simulink model "speed_ctl_tf_sim"  (R2023a)
settings: configuration reference "config" (kept outside this file)
model workspace (MATLAB code in the model file + MAT data in the model file):
  cmdLim = Simulink.Parameter
  cmdLim.Value = 15
  cmdLim.Description = 'Limit for controlling the maximum surface command angle.'
  cmdLim.Min = 0
  cmdLim.Max = 90
  cmdLim.DocUnits = 'deg'
  dispGain = Simulink.Parameter
  dispGain.Value = 0.75
  dispGain.Description = 'Gain applied to the displacement error.'
  dispGain.Min = 0
  dispGain.Max = []
  dispGain.DocUnits = 'deg/sec/deg'
  dispLim = Simulink.Parameter
  dispLim.Value = 30
  dispLim.Description = 'Limit for controlling the maximum commanded angle.'
  dispLim.Min = 0
  dispLim.Max = 180
  dispLim.DocUnits = 'deg'
  intGain = Simulink.Parameter
  intGain.Value = 0.5
  intGain.Description = 'Gain applied to the integral error.'
  intGain.Min = 0
  intGain.Max = []
  intGain.DocUnits = 'deg/sec/deg/sec'
  intLim = Simulink.Parameter
  intLim.Value = 5
  intLim.Description = 'Limit for controlling the maximum commanded angle.'
  intLim.Min = 0
  intLim.Max = 90
  intLim.DocUnits = 'deg'
  rateGain = Simulink.Parameter
  rateGain.Value = 2
  rateGain.Description = 'Gain applied to the rate error.'
  rateGain.Min = 0
  rateGain.Max = []
  rateGain.DocUnits = 'deg/deg/sec'
  rateLim = Simulink.Parameter
  rateLim.Value = 6
  rateLim.Description = 'Limit for controlling the maximum commanded angle.'
  rateLim.Min = 0
  rateLim.Max = 180
  rateLim.DocUnits = 'deg/sec'
  hdgGain = Simulink.Parameter
  hdgGain.Value = 0.015
  b = Simulink.Parameter
  b.Value = 0.001
  b.DataType = 'single'
  b.Complexity = 'real'
  b.Dimensions = [1 1]
  current_ctl_bw_rad_s = Simulink.Parameter
  current_ctl_bw_rad_s.Value = 6666.7
  current_ctl_bw_rad_s.Description = '电流环设计带宽'
  current_ctl_bw_rad_s.DataType = 'single'
  current_ctl_bw_rad_s.Complexity = 'real'
  current_ctl_bw_rad_s.Dimensions = [1 1]
  delta = Simulink.Parameter
  delta.Value = 6
  delta.Description = '速度环阻尼因子'
  delta.DataType = 'double'
  delta.Complexity = 'real'
  delta.Dimensions = [1 1]
  dt = Simulink.Parameter
  dt.Value = 1e-05
  dt.DataType = 'single'
  dt.Complexity = 'real'
  dt.Dimensions = [1 1]
  fc = Simulink.Parameter
  fc.Value = 0.001
  fc.DataType = 'single'
  fc.Complexity = 'real'
  fc.Dimensions = [1 1]
  flux = Simulink.Parameter
  flux.Value = 0.0083
  flux.DataType = 'single'
  flux.Complexity = 'real'
  flux.Dimensions = [1 1]
  fs = Simulink.Parameter
  fs.Value = 10000
  fs.Description = '位置环 速度环执行频率'
  fs.DataType = 'single'
  fs.Complexity = 'real'
  fs.Dimensions = [1 1]
  iq_max = Simulink.Parameter
  iq_max.Value = 30
  iq_max.DataType = 'double'
  iq_max.Complexity = 'real'
  iq_max.Dimensions = [1 1]
  j = Simulink.Parameter
  j.Value = 0.0115
  j.DataType = 'single'
  j.Complexity = 'real'
  j.Dimensions = [1 1]
  j_inv = Simulink.Parameter
  j_inv.Value = 86.9565217391
  j_inv.DataType = 'single'
  j_inv.Complexity = 'real'
  j_inv.Dimensions = [1 1]
  kt = Simulink.Parameter
  kt.Value = 0.05
  kt.Description = '转矩常数 N*M/A'
  kt.DataType = 'single'
  kt.Complexity = 'real'
  kt.Dimensions = [1 1]
  ld = Simulink.Parameter
  ld.Value = 0.00059
  ld.DataType = 'single'
  ld.Complexity = 'real'
  ld.Dimensions = [1 1]
  ld_inv = Simulink.Parameter
  ld_inv.Value = 1694.91525424
  ld_inv.DataType = 'single'
  ld_inv.Complexity = 'real'
  ld_inv.Dimensions = [1 1]
  lq = Simulink.Parameter
  lq.Value = 0.00059
  lq.DataType = 'single'
  lq.Complexity = 'real'
  lq.Dimensions = [1 1]
  lq_inv = Simulink.Parameter
  lq_inv.Value = 1694.91525424
  lq_inv.DataType = 'single'
  lq_inv.Complexity = 'real'
  lq_inv.Dimensions = [1 1]
  pn = Simulink.Parameter
  pn.Value = 4
  pn.DataType = 'single'
  pn.Complexity = 'real'
  pn.Dimensions = [1 1]
  r = Simulink.Parameter
  r.Value = 1.02
  r.DataType = 'single'
  r.Complexity = 'real'
  r.Dimensions = [1 1]
  tc = Simulink.Parameter
  tc.Value = 5e-05
  tc.Description = '电流环运行频率用来设定综合仿真的参数'
  tc.DataType = 'double'
  tc.Complexity = 'real'
  tc.Dimensions = [1 1]
  tp = Simulink.Parameter
  tp.Value = 0.0001
  tp.Description = '位置环速度环执行周期'
  tp.DataType = 'double'
  tp.Complexity = 'real'
  tp.Dimensions = [1 1]
  ts = Simulink.Parameter
  ts.Value = 1e-05
  ts.Description = '模型仿真的周期 s'
  ts.DataType = 'double'
  ts.Complexity = 'real'
  ts.Dimensions = [1 1]
  wn = Simulink.Parameter
  wn.Value = 9434
  wn.DataType = 'double'
  wn.Complexity = 'real'
  wn.Dimensions = [1 1]
undefined symbols (not defined in the file): DiscIntNeverNeededParam
settings Model: RequirementInfo={} %GIDa_fe9045fd_0412_4b6e_8206_617cc20e6fde  DataDictionary=model_config.sldd  ParameterArgumentNames=b,current_ctl_bw_rad_s,dt,fc,flux,fs,j,j_inv,kt,ld,ld_inv,lq,lq_inv,pn,r  Creator=Administrator  LastModifiedBy=Administrator
settings ConfigSetRef: SourceName=config

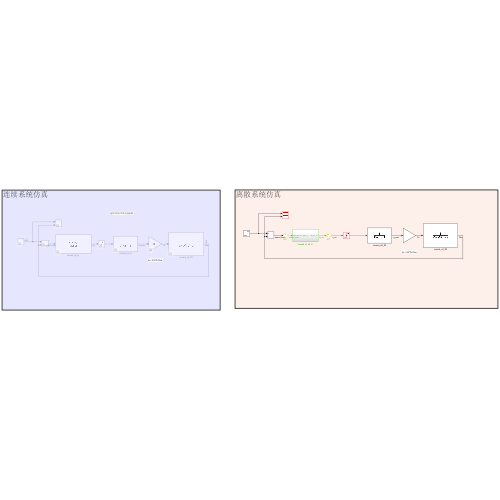
[thumbnail: Simulink's stored preview of the top-level diagram]
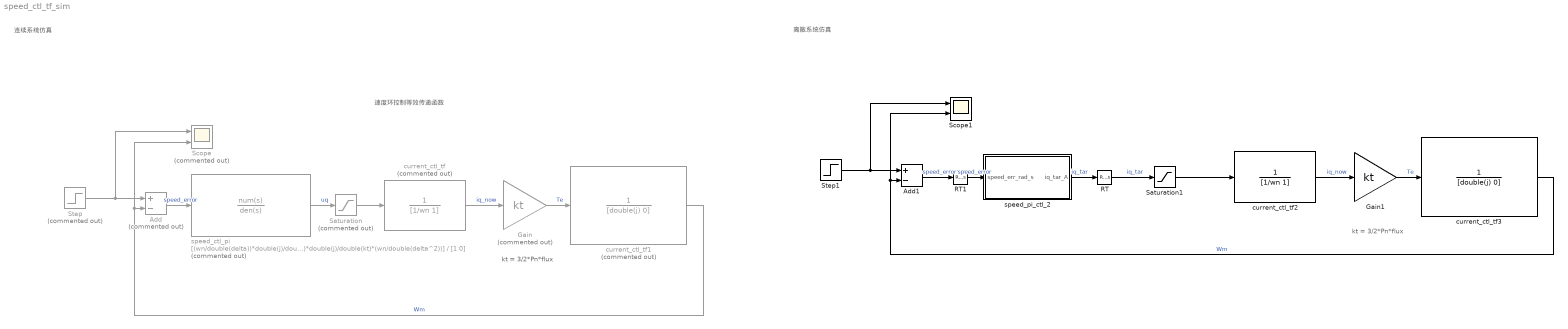
== system speed_ctl_tf_sim ==
  note: 速度环控制等效传递函数
  note: kt = 3/2*Pn*flux
  note: 离散系统仿真
  note: 连续系统仿真
  note: kt = 3/2*Pn*flux
  Add : Sum  Commented=on  Inputs=+-
  Add1 : Sum  Inputs=+-
  Gain : Gain  Commented=on  Gain=kt
  Gain1 : Gain  Gain=kt
  RT : RateTransition  OutPortSampleTime=1e-05
  RT1 : RateTransition  OutPortSampleTime=0.0001
  Saturation : Saturate  Commented=on  UpperLimit=iq_max  LowerLimit=-iq_max
  Saturation1 : Saturate  UpperLimit=iq_max  LowerLimit=-iq_max
  Scope : Scope  Commented=on  NumInputPorts=2
  Scope1 : Scope  NumInputPorts=2
  Step : Step  Commented=on  SampleTime=0
  Step1 : Step  SampleTime=0
  current_ctl_tf : TransferFcn  Commented=on  Denominator=[1/wn 1]
  current_ctl_tf1 : TransferFcn  Commented=on  Denominator=[double(j) 0]
  current_ctl_tf2 : TransferFcn  Denominator=[1/wn 1]
  current_ctl_tf3 : TransferFcn  Denominator=[double(j) 0]
  speed_ctl_pi : TransferFcn  Commented=on  Numerator="[(wn/double(delta))*double(j)/double(kt)    (wn/double(delta))*double(j)/double(kt)*(wn/double(delta^2))]"  Denominator=[1 0]
  speed_pi_ctl_2 : Subsystem  SystemSampleTime=10e-5
  wires:
  current_ctl_tf/1 -> Gain/1  "iq_now"
  Gain/1 -> current_ctl_tf1/1  "Te"
  speed_ctl_pi/1 -> Saturation/1  "uq"
  Add/1 -> speed_ctl_pi/1  "speed_error"
  Step/1 -> Scope/1, Add/1
  current_ctl_tf1/1 -> Scope/2, Add/2  "Wm"
  Step1/1 -> Scope1/1, Add1/1
  current_ctl_tf3/1 -> Scope1/2, Add1/2  "Wm"
  Add1/1 -> RT1/1  "speed_error"
  speed_pi_ctl_2/1(iq_tar_A) -> RT/1  "iq_tar"
  Gain1/1 -> current_ctl_tf3/1  "Te"
  current_ctl_tf2/1 -> Gain1/1  "iq_now"
  RT/1 -> Saturation1/1  "iq_tar"
  RT1/1 -> speed_pi_ctl_2/1(speed_err_rad_s)  "speed_error"
  Saturation/1 -> current_ctl_tf/1
  Saturation1/1 -> current_ctl_tf2/1

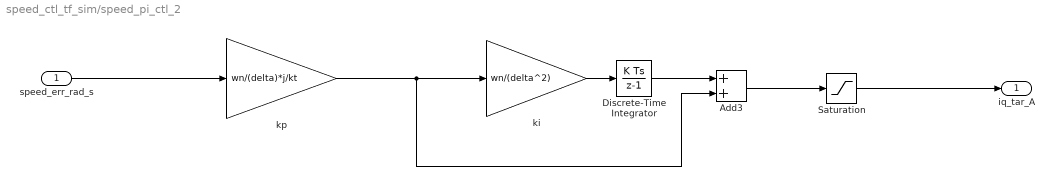
== system speed_ctl_tf_sim/speed_pi_ctl_2 ==
  speed_err_rad_s : Inport
  Add3 : Sum
  Discrete-Time Integrator : DiscreteIntegrator  SampleTime=-1  LimitOutput=on  UpperSaturationLimit=iq_max  LowerSaturationLimit=-iq_max  ICPrevOutput=DiscIntNeverNeededParam  ICPrevScaledInput=DiscIntNeverNeededParam
  Saturation : Saturate  UpperLimit=iq_max  LowerLimit=-iq_max
  ki : Gain  Gain=wn/(delta^2)
  kp : Gain  Gain=wn/(delta)*j/kt
  iq_tar_A : Outport
  wires:
  Add3/1 -> Saturation/1
  Discrete-Time Integrator/1 -> Add3/1
  ki/1 -> Discrete-Time Integrator/1
  kp/1 -> ki/1, Add3/2
  speed_err_rad_s/1 -> kp/1
  Saturation/1 -> iq_tar_A/1
